simulink model "simulink2"  (R2020a)
settings: Solver=ode45  StartTime=0.0  StopTime=100  RelTol=1e-3
settings Model: Creator=16002  LastModifiedBy=16002

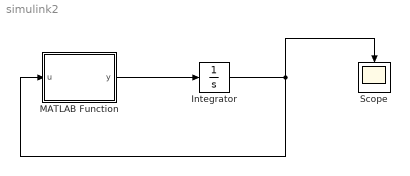
== system simulink2 ==
  Integrator : Integrator  InitialCondition=[-0.2;0.1;0.2]  IgnoreLimit=on
  MATLAB Function : MATLAB Function  TreatAsAtomicUnit=on
  Scope : Scope
  wires:
  Integrator/1 -> MATLAB Function/1(u), Scope/1
  MATLAB Function/1(y) -> Integrator/1

== matlab function simulink2/MATLAB Function ==
  data: u input; y output
function y = fcn(u)
x1=u(1);
x2=u(2);
x3=u(3);
dx1=9*( x2 - ( (2*x1)/7 + (-3*(abs(x1+1)-abs(x1-1)))/14) );
dx2=x1-x2+x3;
dx3=-14.28*x2;
y=[dx1;dx2;dx3]
